simulink library "Collector_Unglazed"  (R2013b)
settings: Solver=ode45  StartTime=0.0  StopTime=10.0  RelTol=1e-3
libraries: carnot x5
settings Model: Creator=lena.frank  LastModifiedBy=drhf

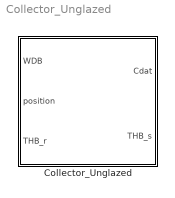
== system Collector_Unglazed ==
  Collector_Unglazed : Subsystem  mask(Unglazed flat plate collector){acol=2.33, len=5, fta=0.9, e_sky=0.9, uc0=10, uc1=3, uc0loss=4, uc1loss=1.5, uc0gain=6, uc1gain=1.5, uc1eta0=0.01, hi=100, c_abs=1e4, c_fl=1e2, lin=0, qua=0, tini=20, nodes=2}
      mask prompts: acol "collector surface (aperture) in [m²]"; len "length between inlet and outlet [m]"; fta "absorption coefficient of the absorber [-]"; e_sky "e thermal emissivity of the absorber (0..1)"; uc0 "U0C heat transfer for condensation [W/(m²*K)]"; uc1 "U1C wind dependent heat transfer for condensation [W/(m²*K*m/s)]"; uc0loss "U0L heat transfer for losses [W/(m²*K)]"; uc1loss "U1L wind dependent heat transfer for losses [W/(m²*K*m/s)]"; uc0gain "U0G heat transfer for gains [W/(m²*K)]"; uc1gain "U1G wind dependent heat transfer for gains [W/(m²*K*m/s)]"; uc1eta0 "U1E wind dependancy of optical efficiency in W/(m²*m/s)"; hi "HI heat transfer between collector and tube [W/(m2.K)]"; c_abs "effective heat capacity of absorber [J/(m²*K)]"; c_fl "effective heat capacity of fluid [J/(m²*K)]"; lin "linear pressure drop in Pa/(kg/s)"; qua "quadratic pressure drop in Pa/(kg/s)²"; tini "initial temperature [degree centigrade]"; nodes "number of nodes (>=2)"
      mask help:
      | 2xN-nodes model:
      | c_abs*dTp/dt=qdot_solar-qdot_conv_gain-qdot_conv_loss-qdot_cond
      |             -qdot_sky-qdot_fluid
      | qdot_solar = absorbed_solar_radiation - U1E*Iglb*vwind
      | qdot_conv_gain = fconv * (U0G + U1G*vwind)*(Tp - Tamb)
      | qdot_conv_loss = (1-fconv)*(U0L + U1L*vwind)*(Tp - Tamb)
      | qdot_cond = fcond*(U0C + U1C*vwind)*ccond*(ps(Tdew) - ps(Tp))
      | qdot_sky = e * const_sigma*(Tp^4 - Tsky^4)
      | qdot_fluid = HI*(Tp-Tfluid)
      | fconv = 1 if Tp > Tamb, 0 otherwise
      | fcond = 1 if Tp below dewpoint, 0 otherwise
      | Look under mask to change the incidence angle modifier, the pressure drop and the radiation calculation method.
      mask init:
      | acol = max(acol, 0.01);
      | fta = max(fta,0);
      | inv_c_abs = 1/max(c_abs,1);
      | inv_c_fl = 1/max(c_fl,1);
      mask Help: web(fullfile(path_carnot('help'),'Collector_Unglazed.html'),'-helpbrowser')
      mask Display: plot(-30,-30,130,120,[0,70,70,0,0],[-0,-0,5,5,-0],[30,30,100,100,30],[100,94,94,100,100],[32,1],[94,5],[40,10],[94,5],[49,19],[94,5],[57,27],[94,5],[65,35],[94,5],[73,43],[94,5],[82,51],[94,5],[90,60],[94,5],[98,68],[94,5])

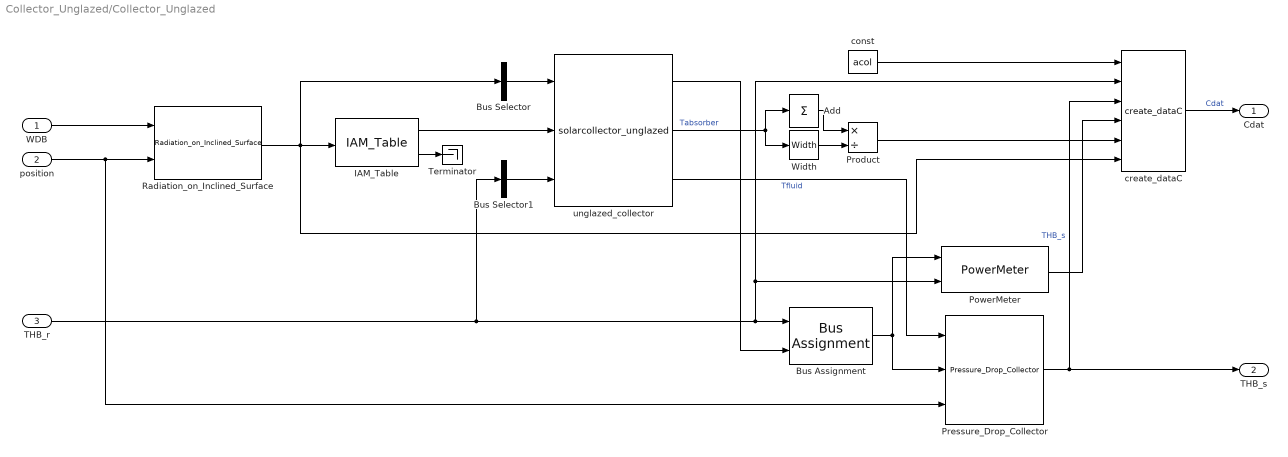
== system Collector_Unglazed/Collector_Unglazed ==
  WDB : Inport
  position : Inport  Port=2
  THB_r : Inport  Port=3
  Add : Sum  Inputs=1
  Bus Assignment : BusAssignment  AssignedSignals=Temperature
  Bus Selector : BusSelector  OutputSignals=Solar_Radiation_direct_surface,Solar_Radiation_diffuse_surface,Temperature_Ambient,Temperature_Sky_Radiation,Relative_Humidity,Station_Pressure,Wind_Speed  OutputAsBus=on
  Bus Selector1 : BusSelector  OutputSignals=Temperature,MassFlow,Pressure,FluidType,FluidMix  OutputAsBus=on
  IAM_Table : carnot/Source/Solar_Thermal/IncidenceAngleModifier/IAM_Table  fta=0.9  angle=[0:5:90]  Kb="[1.0000    1.0000    0.9999    0.9996    0.9991    0.9982    0.9965  0.9935    0.9886    0.9807    0.9678    0.9473    0.9148    0.8638   0.7846    0.6644    0.4907    0.2599    0.0000]"  Kd=0.92
  PowerMeter : carnot/Control/PowerMeter
  Pressure_Drop_Collector : carnot/Basic/Pressure_Drop/Pressure_Drop_Collector  len=len  lin=lin  qua=qua
  Product : Product  Inputs=*/  RndMeth=Zero
  Radiation_on_Inclined_Surface : carnot/Weather/Radiation_on_Inclined_Surface  sky=Perez 1990  reflect=0.2
  Terminator : Terminator
  Width : Width
  const : Constant  Value=acol
  create_dataC : carnot/Source/Solar_Thermal/Collector_EN12975/create_dataC
  unglazed_collector : S-Function  FunctionName=solarcollector_unglazed  Parameters=acol, uc0, uc1, uc0loss, uc1loss, uc0gain, uc1gain, e_sky, uc1eta0, hi, inv_c_abs, inv_c_fl, len, tini, nodes  EnableBusSupport=off
  Cdat : Outport
  THB_s : Outport  Port=2
  wires:
  IAM_Table/1 -> unglazed_collector/2
  Bus Assignment/1 -> Pressure_Drop_Collector/2, PowerMeter/1
  Radiation_on_Inclined_Surface/1 -> Bus Selector/1, create_dataC/6, IAM_Table/1
  position/1 -> Pressure_Drop_Collector/3, Radiation_on_Inclined_Surface/2
  WDB/1 -> Radiation_on_Inclined_Surface/1
  THB_r/1 -> Bus Selector1/1, Bus Assignment/1, create_dataC/2, PowerMeter/2
  Bus Selector/1 -> unglazed_collector/1
  Bus Selector1/1 -> unglazed_collector/3
  IAM_Table/2 -> Terminator/1
  unglazed_collector/1 -> Bus Assignment/2
  unglazed_collector/2 -> Add/1, Width/1  "Tabsorber"
  const/1 -> create_dataC/1
  create_dataC/1 -> Cdat/1  "Cdat"
  PowerMeter/1 -> create_dataC/4
  Add/1 -> Product/1
  Product/1 -> create_dataC/5
  Width/1 -> Product/2
  Pressure_Drop_Collector/1 -> create_dataC/3, THB_s/1  "THB_s"
  unglazed_collector/3 -> Pressure_Drop_Collector/1  "Tfluid"
